simulink model "BallOnBeam_model"  (R2018b)
settings: Solver=FixedStepAuto  StartTime=0.0  StopTime=10.0  FixedStep=1e-3  RelTol=1e-3
values from neighbouring files (symbols this model uses):
  g = 9.81    [Main.m]
  K = 0.0275    [Main.m]
  m = p_steel*Vball    (= 29.1393220081)    [Main.m]
  R = 5    [Main.m]
  u0 = 0    [Main.m]
  x10 = 0    [Main.m]
  x20 = 0    [Main.m]
  x30 = 0    [Main.m]
  x40 = 0    [Main.m]
libraries: vrlib x3
settings Model: Creator=Eduardo  LastModifiedBy=ohara

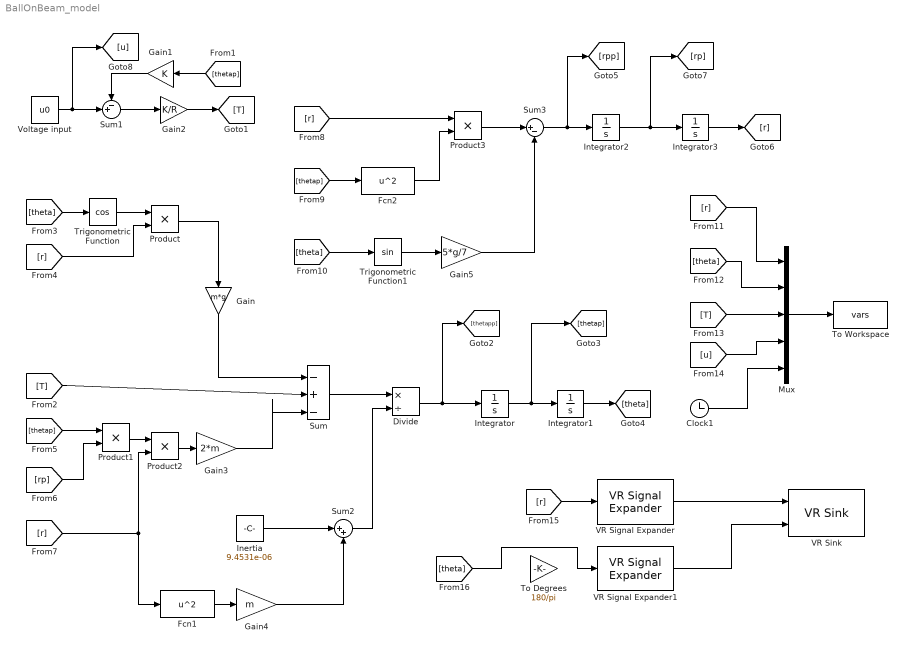
== system BallOnBeam_model ==
  Clock1 : Clock
  Divide : Product  Inputs=*/
  Fcn1 : Fcn  Expr=u^2
  Fcn2 : Fcn  Expr=u^2
  Gain : Gain  Gain=m*g
  Gain1 : Gain  Gain=K
  Gain2 : Gain  Gain=K/R
  Gain3 : Gain  Gain=2*m
  Gain4 : Gain  Gain=m
  Gain5 : Gain  Gain=5*g/7
  Inertia : Constant  Value=9.4531e-06
  Integrator : Integrator  InitialCondition=x30
  Integrator1 : Integrator  InitialCondition=x10
  Integrator2 : Integrator  InitialCondition=x40
  Integrator3 : Integrator  InitialCondition=x20
  Mux : Mux  Inputs=5
  Product{,1..3} (4 alike) : Product
  Sum : Sum  Inputs=-+-|
  Sum1 : Sum  Inputs=-+|
  Sum2 : Sum  Inputs=|++
  Sum3 : Sum  Inputs=|+-
  "To Degrees " : Gain  Gain=180/pi
  To Workspace : ToWorkspace  VariableName=vars  SaveFormat=Timeseries  SampleTime=-1
  Trigonometric Function : Trigonometry  Operator=cos
  Trigonometric Function1 : Trigonometry
  VR Signal Expander : vrlib/VR Signal Expander  outwidth=3  outidx=[1]
      settings: SourceProductName=Simulink 3D Animation  SourceProductBaseCode=VR
  VR Signal Expander1 : vrlib/VR Signal Expander  outwidth=4  outidx=[4 3]
      settings: SourceProductName=Simulink 3D Animation  SourceProductBaseCode=VR
  VR Sink : vrlib/VR Sink  InstantiateOnLoad=on  SampleTime=0.01  ViewEnable=on  RemoteChange=off  RemoteView=off  FieldsWritten=Ball.translation.3.1.1.double#Rod.rotation.4.1.1.double  WorldFileName=ballonbeam_3danim.WRL  AutoView=off  VideoDimensions=[]  AllowVariableSize=off
      settings: SourceProductBaseCode=VR
  "Voltage input " : Constant  Value=u0
  wires:
  Gain/1 -> Sum/1
  [T] -> Sum/2
  "Voltage input "/1 -> [u], Sum1/2
  Gain1/1 -> Sum1/1
  Sum1/1 -> Gain2/1
  [thetap] -> Gain1/1
  Gain2/1 -> [T]
  [theta] -> Trigonometric Function/1
  Trigonometric Function/1 -> Product/1
  [r] -> Product/2
  Product/1 -> Gain/1
  [thetap] -> Product1/1
  [rp] -> Product1/2
  Product1/1 -> Product2/1
  [r] -> Fcn1/1, Product2/2
  Product2/1 -> Gain3/1
  Gain3/1 -> Sum/3
  Sum/1 -> Divide/1
  Inertia/1 -> Sum2/1
  Fcn1/1 -> Gain4/1
  Gain4/1 -> Sum2/2
  Sum2/1 -> Divide/2
  Divide/1 -> [thetapp], Integrator/1
  Integrator/1 -> [thetap], Integrator1/1
  Integrator1/1 -> [theta]
  [r] -> Product3/1
  Fcn2/1 -> Product3/2
  [thetap] -> Fcn2/1
  Product3/1 -> Sum3/1
  [theta] -> Trigonometric Function1/1
  Trigonometric Function1/1 -> Gain5/1
  Gain5/1 -> Sum3/2
  Sum3/1 -> [rpp], Integrator2/1
  Integrator2/1 -> [rp], Integrator3/1
  Integrator3/1 -> [r]
  Mux/1 -> To Workspace/1
  [r] -> Mux/1
  [theta] -> Mux/2
  Clock1/1 -> Mux/5
  [T] -> Mux/3
  [u] -> Mux/4
  [r] -> VR Signal Expander/1
  VR Signal Expander/1 -> VR Sink/1
  VR Signal Expander1/1 -> VR Sink/2
  [theta] -> VR Signal Expander1/1
